simulink model "task2"  (R2023b)
settings: Solver=VariableStepAuto  StartTime=0.0  StopTime=10.0  RelTol=1e-3

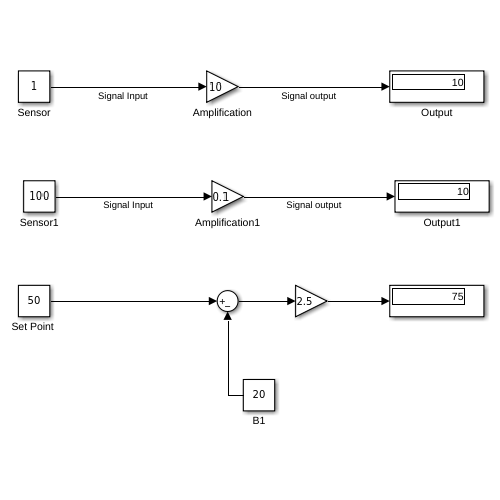
[thumbnail: Simulink's stored preview of the top-level diagram]
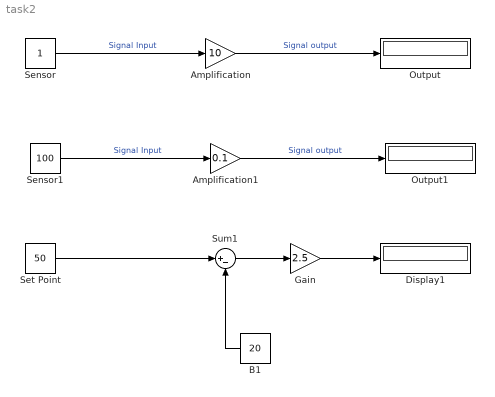
== system task2 ==
  Amplification : Gain  Gain=10
  Amplification1 : Gain  Gain=0.1
  B1 : Constant  Value=20
  Display1 : Display
  Gain : Gain  Gain=2.5
  Output : Display
  Output1 : Display
  Sensor : Constant
  Sensor1 : Constant  Value=100
  "Set Point " : Constant  Value=50
  Sum1 : Sum  Inputs=|+-
  wires:
  "Set Point "/1 -> Sum1/1
  B1/1 -> Sum1/2
  Sensor/1 -> Amplification/1  "Signal Input"
  Amplification/1 -> Output/1  "Signal output"
  Gain/1 -> Display1/1
  Sum1/1 -> Gain/1
  Amplification1/1 -> Output1/1  "Signal output"
  Sensor1/1 -> Amplification1/1  "Signal Input"
